simulink model "simulation_3d_line_new"  (R2015a)
settings: Solver=ode45  StartTime=0.0  StopTime=5  RelTol=1e-3
settings Model: Creator=Παναγιώτης Κυριάκης  LastModifiedBy=Παναγιώτης Κυριάκης

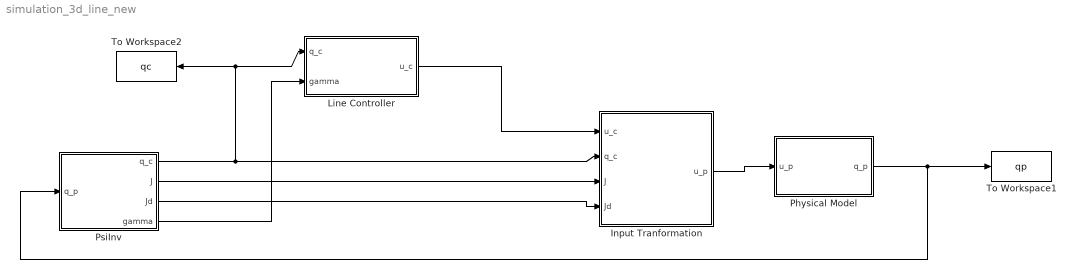
== system simulation_3d_line_new ==
  "Input Tranformation " : MATLAB Function  TreatAsAtomicUnit=on
  Line Controller : MATLAB Function  TreatAsAtomicUnit=on
  Physical Model : Subsystem
  PsiInv : MATLAB Function  TreatAsAtomicUnit=on
  To Workspace1 : ToWorkspace  VariableName=qp  SaveFormat=Timeseries  SampleTime=-1
  To Workspace2 : ToWorkspace  VariableName=qc  SaveFormat=Timeseries  SampleTime=-1
  wires:
  Line Controller/1(u_c) -> "Input Tranformation "/1(u_c)
  "Input Tranformation "/1(u_p) -> Physical Model/1(u_p)
  Physical Model/1(q_p) -> PsiInv/1(q_p), To Workspace1/1
  PsiInv/1(q_c) -> To Workspace2/1, Line Controller/1(q_c), "Input Tranformation "/2(q_c)
  PsiInv/2(J) -> "Input Tranformation "/3(J)
  PsiInv/3(Jd) -> "Input Tranformation "/4(Jd)
  PsiInv/4(gamma) -> Line Controller/2(gamma)

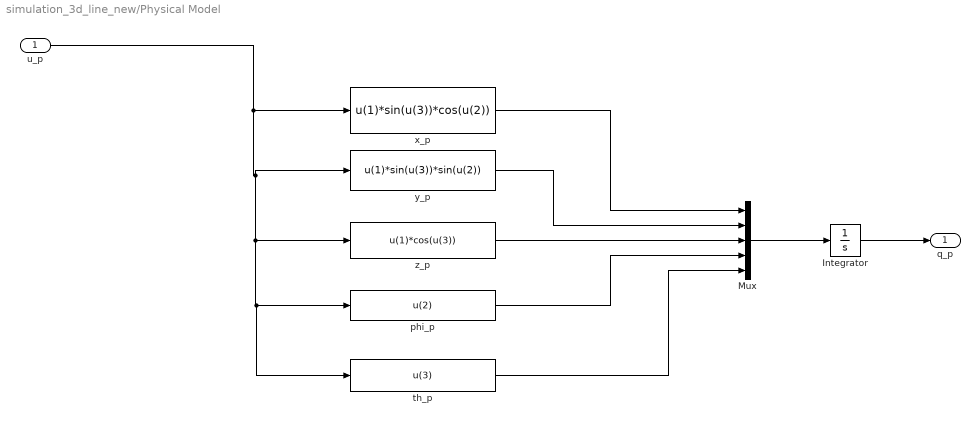
== system simulation_3d_line_new/Physical Model ==
  u_p : Inport
  Integrator : Integrator  InitialCondition=[9 -0.8 -0.5 pi/2 pi/9]  UpperSaturationLimit=1000  LowerSaturationLimit=-1000
  Mux : Mux  Inputs=5
  phi_p : Fcn  Expr=u(2)
  th_p : Fcn  Expr=u(3)
  "x_p " : Fcn  Expr=u(1)*sin(u(3))*cos(u(2))
  y_p : Fcn  Expr=u(1)*sin(u(3))*sin(u(2))
  z_p : Fcn  Expr=u(1)*cos(u(3))
  q_p : Outport
  wires:
  y_p/1 -> Mux/2
  z_p/1 -> Mux/3
  th_p/1 -> Mux/5
  Integrator/1 -> q_p/1
  "x_p "/1 -> Mux/1
  phi_p/1 -> Mux/4
  Mux/1 -> Integrator/1
  u_p/1 -> th_p/1, phi_p/1, z_p/1, y_p/1, "x_p "/1

== matlab function simulation_3d_line_new/PsiInv ==
  data: q_p input; q_c output; J output; Jd output; gamma output
function [q_c, J, Jd, gamma]  = PsiInv(q_p)
     
    % Find canonical cordinates
    xc = 10*log(q_p(1)/10);
    yc = q_p(2)-sin(xc);
    zc = q_p(3)-cos(xc);
    
    % Find transformation Jacobian and its Derivative wrt to xc
    J = [exp(0.1*xc) 0 0; 
         cos(xc) 1 0;
        -sin(xc) 0 1];
    Jd = [0.1*exp(0.1*xc) 0 0; 
          -sin(xc) 0 0;
          -cos(xc) 0 0];
      
    % Get physical angles and their unit vector
    th_p = q_p(5);
    phi_p = q_p(4);
    
    cp = [sin(th_p)*cos(phi_p);
          sin(th_p)*sin(phi_p);
          cos(th_p)];

      
    % Find canonical phi, th   
    cc = J\cp/norm(J\cp);    
    phi_c = atan2(cc(2),cc(1));
    th_c = acos(cc(3));
    
    % Canonical state vector
    q_c =[  xc;
            yc;
            zc;
            phi_c;
            th_c];   
    % calculate gamma);
    gamma = sqrt(cc'*(J'*J)*cc);
end

== matlab function simulation_3d_line_new/Input Tranformation  ==
  data: u_c input; q_c input; J input; u_p output; Jd input
function u_p = M(u_c,q_c,J,Jd)
    
    % Initialization
    C = zeros(2,3);
    D = eye(2);
    M = eye(3);
    
    % Construct needed elements of Cartesian tensor
    e12=[1 0 0]'*[0 1 0];
    e21=[0 1 0]'*[1 0 0];
    e33=[0 0 1]'*[0 0 1];
    
    % Get canonical angles
    th_c = q_c(5);
    phi_c = q_c(4);    
    
    % Construct the vector cc and its derivatives
    cc = [sin(th_c)*cos(phi_c);sin(th_c)*sin(phi_c);cos(th_c)];
    cc_phi_c = [-sin(th_c)*sin(phi_c);sin(th_c)*cos(phi_c);0];
    cc_th_c = [cos(th_c)*cos(phi_c);cos(th_c)*sin(phi_c);-sin(th_c)];
    
    % Find the length ratio
    gamma = sqrt(cc'*J'*J*cc);
    % Find the coefficients appearing in C,D
    Aphi = cc'*J'*(e12-e21)/(gamma^2-cc'*J'*e33*J*cc);
    Ath = -gamma*[0 0 1]/sqrt(gamma^2-cc'*J'*e33*J*cc);
    % Find C
    C(1,1) = Aphi*Jd*cc;
    C(2,1) = Ath*(2*(gamma^2)*Jd-cc'*(Jd'*J+J'*Jd)*cc*J)*cc/(2*gamma^3);
 
    % Find D
    D(1,1) = Aphi*J*cc_phi_c;
    D(1,2) = Aphi*J*cc_th_c;
    D(2,1) = Ath*J*(cc_phi_c*(cc')-cc*(cc_phi_c'))*(J')*J*cc/gamma^3;
    D(2,2) = Ath*J*(cc_th_c*(cc')-cc*(cc_th_c'))*(J')*J*cc/gamma^3;
    % Find M
    
    M(1,1) = gamma;
    M(2:3,1) = C*cc;
    M(2:3,2:3) = D;

    % Transform the control
    u_p = M*u_c;

 end

== matlab function simulation_3d_line_new/Line Controller ==
  data: q_c input; u_c output; gamma input
function u_c = LineCon(q_c,gamma)
 
    K2 = -20*[1;0;0]; 
    V=4;
    r_c = [0; q_c(2); q_c(3)];
        
    v = -1000*r_c - K2;

    v=V*v/norm(v);
    
    
    u_c = [ V/gamma; 
            atan2(v(2),v(1));
            acos(v(3)/V)];    

end
